simulink model "BPSK_Demod_OpenLoopClkRec_Prototype"  (R2013a)
settings: Solver=ode3  SolverMode=SingleTasking  StartTime=0.0  StopTime=10000/1200  FixedStep=1/480e3  RelTol=1e-3
undefined symbols (not defined in the file or in its folder): DiscIntNeverNeededParam
libraries: dsparch4 x9, simulink_extras x7, commsynccomp2 x6, dspsigops x6, simulink x5, commsink2 x2, commchan3 x1, commrflib2 x1, commrandsrc2 x1
settings Model: Creator=tibbs2010  LastModifiedBy=Cedric
settings DataIOCC: SignalLoggingSaveFormat=ModelDataLogs
settings DebuggingCC: MultiTaskDSMMsg=warning  MultiTaskCondExecSysMsg=none  StrictBusMsg=None
settings RTWCC: IncludeERTFirstTime=on

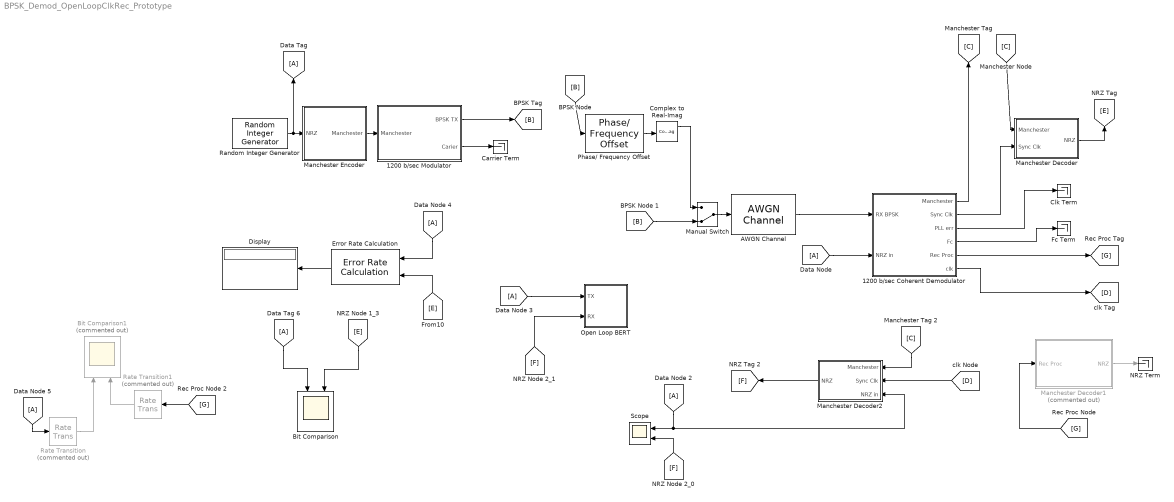
== system BPSK_Demod_OpenLoopClkRec_Prototype ==
  1200 b/sec Modulator : Subsystem
  1200 b/sec Coherent Demodulator : Subsystem
  AWGN Channel : commchan3/AWGN Channel  InputProcessing=Columns as channels (frame based)  seed=randseed  noiseMode="Signal to noise ratio  (Eb/No)"  EbNodB=0  EsNodB=10  SNRdB=10  bitsPerSym=1  Ps=12.5  Tsym=1/1200  variance=1
  Bit Comparison : Scope  NumInputPorts=2
      settings: YMin=-0.5~-0.5  YMax=1.5~1.5
  Bit Comparison1 : Scope  Commented=on  NumInputPorts=2
      settings: YMin=-0.5~-0.5  YMax=1.5~1.5  SaveName=ScopeData19
  Carrier Term : Terminator
  Clk Term : Terminator
  Complex to Real-Imag : ComplexToRealImag
  Display : Display
  Error Rate Calculation : commsink2/Error Rate Calculation  N=3  st_delay=0  cp_mode=Entire frame  subframe=[]  PMode=Port  WsName=ErrorVec  RsMode2=off  stop=off  numErr=100  maxBits=1e6
  Fc Term : Terminator
  Manchester Encoder : Subsystem
  Manchester Decoder : Subsystem
  Manchester Decoder1 : Subsystem  Commented=on
  Manchester Decoder2 : Subsystem
  Manual Switch : ManualSwitch  CurrentSetting=0
  NRZ Term : Terminator
  Open Loop BERT : Subsystem
  Phase/ Frequency Offset : commrflib2/Phase// Frequency Offset  phaseOffset=30  freqPort=off  freqOffset=0
  Random Integer Generator : commrandsrc2/Random Integer Generator  mul=2  seed=randseed  Ts=1/1200  frameBased=off  sampPerFrame=1  orient=off  outDataType=double
  Rate Transition : RateTransition  Commented=on  OutPortSampleTime=1/1200
  Rate Transition1 : RateTransition  Commented=on  OutPortSampleTime=1/1200
  Scope : Scope  NumInputPorts=2
      settings: YMin=-5~-5  YMax=5~5  SaveName=ScopeData26
  wires:
  Error Rate Calculation/1 -> Display/1
  1200 b/sec Coherent Demodulator/1(Manchester) -> [C]
  1200 b/sec Coherent Demodulator/2(Sync Clk) -> Manchester Decoder/2(Sync Clk)
  Phase/ Frequency Offset/1 -> Complex to Real-Imag/1
  Complex to Real-Imag/1 -> Manual Switch/1
  Manual Switch/1 -> AWGN Channel/1
  AWGN Channel/1 -> 1200 b/sec Coherent Demodulator/1(RX BPSK)
  1200 b/sec Coherent Demodulator/5(Rec Proc) -> [G]
  1200 b/sec Coherent Demodulator/3(PLL err) -> Clk Term/1
  1200 b/sec Coherent Demodulator/4(Fc) -> Fc Term/1
  Rate Transition/1 -> Bit Comparison1/1
  Rate Transition1/1 -> Bit Comparison1/2
  1200 b/sec Coherent Demodulator/6(clk) -> [D]
  [A] -> Open Loop BERT/1(TX)
  [B] -> Phase/ Frequency Offset/1
  [B] -> Manual Switch/2
  [A] -> 1200 b/sec Coherent Demodulator/2(NRZ in)
  [A] -> Rate Transition/1
  [A] -> Manchester Decoder2/3(NRZ in), Scope/1
  [A] -> Error Rate Calculation/1
  [A] -> Bit Comparison/1
  [C] -> Manchester Decoder/1(Manchester)
  [C] -> Manchester Decoder2/1(Manchester)
  [D] -> Manchester Decoder2/2(Sync Clk)
  Manchester Decoder/1(NRZ) -> [E]
  [E] -> Bit Comparison/2
  Manchester Decoder2/1(NRZ) -> [F]
  [G] -> Manchester Decoder1/1(Rec Proc)
  [G] -> Rate Transition1/1
  Manchester Decoder1/1(NRZ) -> NRZ Term/1
  [F] -> Open Loop BERT/2(RX)
  [F] -> Scope/2
  [E] -> Error Rate Calculation/2
  1200 b/sec Modulator/2(Carier) -> Carrier Term/1
  1200 b/sec Modulator/1(BPSK TX) -> [B]
  Random Integer Generator/1 -> Manchester Encoder/1(NRZ), [A]
  Manchester Encoder/1(Manchester) -> 1200 b/sec Modulator/1(Manchester)

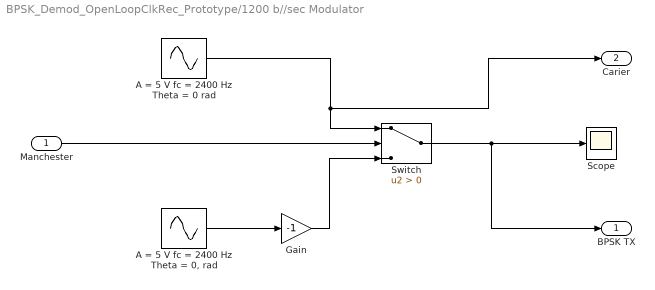
== system BPSK_Demod_OpenLoopClkRec_Prototype/1200 b//sec Modulator ==
  Manchester : Inport
  A = 5 V fc = 2400 Hz Theta = 0 rad : Sin  Amplitude=5  Frequency=2*pi*2400  Phase=pi/2  SampleTime=1/480e3
  "A = 5 V fc = 2400 Hz Theta = 0, rad" : Sin  Amplitude=5  Frequency=2*pi*2400  Phase=pi/2  SampleTime=1/480e3  Offset=pi
  Gain : Gain  Gain=-1
  Scope : Scope
      settings: SaveName=ScopeData22
  Switch : Switch  Criteria=u2 > Threshold
  BPSK TX : Outport
  Carier : Outport  Port=2
  wires:
  A = 5 V fc = 2400 Hz Theta = 0 rad/1 -> Switch/1, Carier/1
  "A = 5 V fc = 2400 Hz Theta = 0, rad"/1 -> Gain/1
  Gain/1 -> Switch/3
  Manchester/1 -> Switch/2
  Switch/1 -> Scope/1, BPSK TX/1

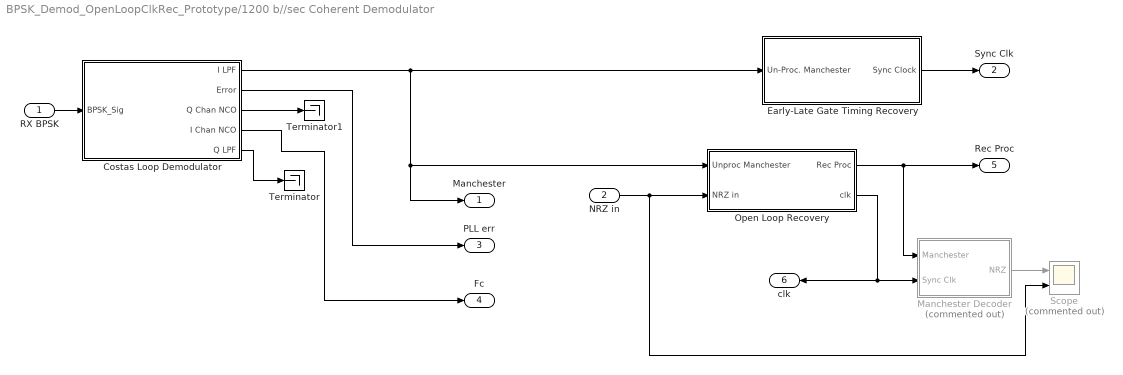
== system BPSK_Demod_OpenLoopClkRec_Prototype/1200 b//sec Coherent Demodulator ==
  RX BPSK : Inport
  NRZ in : Inport  Port=2
  Costas Loop Demodulator : Subsystem
  Early-Late Gate Timing Recovery : Subsystem
  Manchester Decoder : Subsystem  Commented=on
  Open Loop Recovery : Subsystem
  Scope : Scope  Commented=on  NumInputPorts=2
      settings: YMin=-5~-5  YMax=5~5  SaveName=ScopeData20
  Terminator : Terminator
  Terminator1 : Terminator
  Manchester : Outport
  Sync Clk : Outport  Port=2
  PLL err : Outport  Port=3
  Fc : Outport  Port=4
  Rec Proc : Outport  Port=5
  clk : Outport  Port=6
  wires:
  RX BPSK/1 -> Costas Loop Demodulator/1(BPSK_Sig)
  Early-Late Gate Timing Recovery/1(Sync Clock) -> Sync Clk/1
  Costas Loop Demodulator/2(Error) -> PLL err/1
  Costas Loop Demodulator/4(I Chan NCO) -> Fc/1
  Costas Loop Demodulator/1(I LPF) -> Manchester/1, Open Loop Recovery/1(Unproc Manchester), Early-Late Gate Timing Recovery/1(Un-Proc. Manchester)
  Open Loop Recovery/1(Rec Proc) -> Rec Proc/1, Manchester Decoder/1(Manchester)
  NRZ in/1 -> Scope/2, Open Loop Recovery/2(NRZ in)
  Open Loop Recovery/2(clk) -> Manchester Decoder/2(Sync Clk), clk/1
  Manchester Decoder/1(NRZ) -> Scope/1
  Costas Loop Demodulator/3(Q Chan NCO) -> Terminator1/1
  Costas Loop Demodulator/5(Q LPF) -> Terminator/1

== system BPSK_Demod_OpenLoopClkRec_Prototype/Manchester Encoder ==
  NRZ : Inport
  Logical Operator : Logic  Operator=XOR  IconShape=distinctive  AllPortsSameDT=off  OutDataTypeStr=boolean
  Rate Transition : RateTransition  OutPortSampleTime=1/480e3
  TX Clk : DiscretePulseGenerator  PulseType=Time based  Period=1/1200  PulseWidth=50
  Manchester : Outport
  wires:
  Rate Transition/1 -> Logical Operator/1
  Logical Operator/1 -> Manchester/1
  NRZ/1 -> Rate Transition/1
  TX Clk/1 -> Logical Operator/2

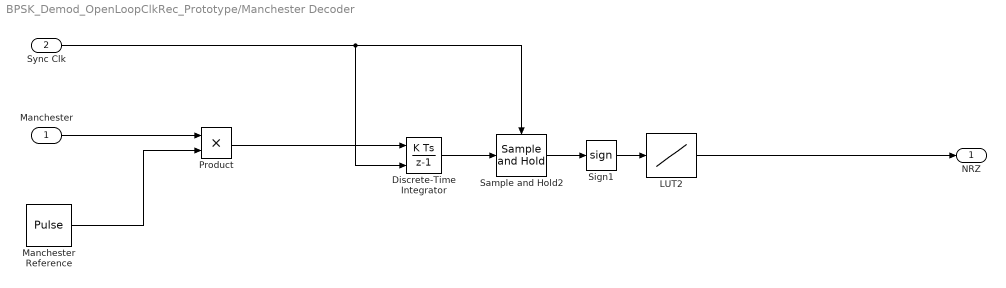
== system BPSK_Demod_OpenLoopClkRec_Prototype/Manchester Decoder ==
  Manchester : Inport
  Sync Clk : Inport  Port=2
  Discrete-Time Integrator : DiscreteIntegrator  ExternalReset=rising  SampleTime=1/480e3  ICPrevOutput=DiscIntNeverNeededParam  ICPrevScaledInput=DiscIntNeverNeededParam
  LUT2 : Lookup_n-D  NumberOfTableDimensions=1  BreakpointsForDimension1=[-1 0 1]  Table=[0 0 1]  RndMeth=Simplest  InputSameDT=on
  Manchester Reference : DiscretePulseGenerator  PulseType=Time based  Period=1/1200  PulseWidth=50  PhaseDelay=(1/1200)/2
  Product : Product
  Sample and Hold2 : dspsigops/Sample and Hold  trig=Falling edge  initCond=0  latchinput=off
  Sign1 : Signum
  NRZ : Outport
  wires:
  Discrete-Time Integrator/1 -> Sample and Hold2/1
  Sample and Hold2/1 -> Sign1/1
  Sign1/1 -> LUT2/1
  Manchester/1 -> Product/1
  Product/1 -> Discrete-Time Integrator/1
  LUT2/1 -> NRZ/1
  Sync Clk/1 -> Discrete-Time Integrator/2, Sample and Hold2/Trigger
  Manchester Reference/1 -> Product/2

== system BPSK_Demod_OpenLoopClkRec_Prototype/Manchester Decoder1 ==
  Rec Proc : Inport
  CDR : Subsystem
  ML decoder : Subsystem
  Scope : Scope  NumInputPorts=2
      settings: YMin=-0.5~-5  YMax=1.5~5  SaveName=ScopeData7
  Scope1 : Scope
      settings: YMin=-0.5  YMax=1.5  SaveName=ScopeData9
  NRZ : Outport
  wires:
  CDR/1(CLK) -> Scope/2, ML decoder/1(CLK)
  Rec Proc/1 -> ML decoder/2(Manchester), Scope/1, CDR/1(Edges)
  ML decoder/1(NRZ) -> NRZ/1, Scope1/1

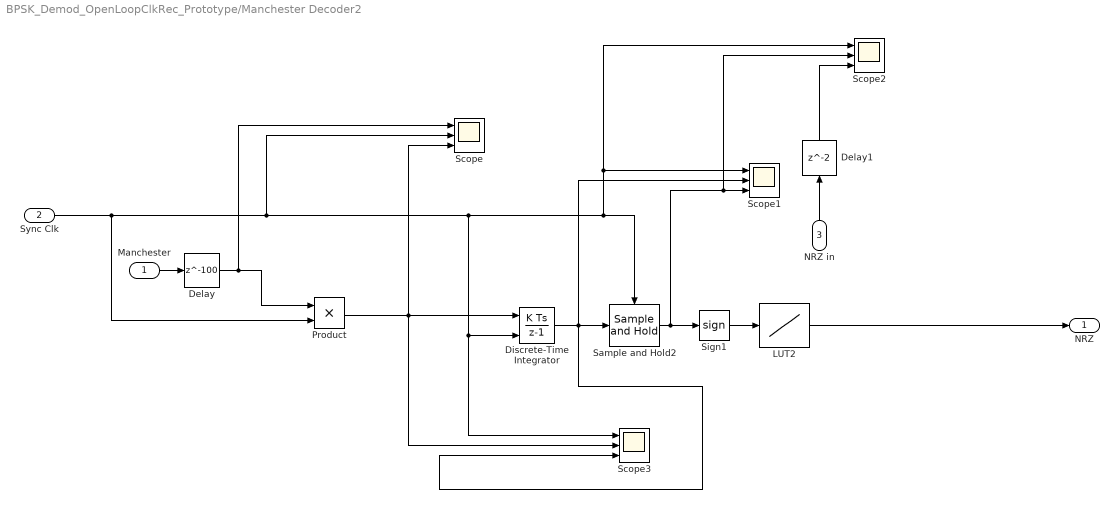
== system BPSK_Demod_OpenLoopClkRec_Prototype/Manchester Decoder2 ==
  Manchester : Inport
  Sync Clk : Inport  Port=2
  NRZ in : Inport  Port=3
  Delay : Delay  DelayLength=100  InitialCondition=0  SampleTime=1/480e3
  Delay1 : Delay  InitialCondition=0  SampleTime=1/1200
  Discrete-Time Integrator : DiscreteIntegrator  ExternalReset=rising  SampleTime=1/480e3  ICPrevOutput=DiscIntNeverNeededParam  ICPrevScaledInput=DiscIntNeverNeededParam
  LUT2 : Lookup_n-D  NumberOfTableDimensions=1  BreakpointsForDimension1=[-1 0 1]  Table=[1 1 0]  RndMeth=Simplest  InputSameDT=on
  Product : Product
  Sample and Hold2 : dspsigops/Sample and Hold  trig=Falling edge  initCond=0  latchinput=off
  Scope{,1..3} (4 alike) : Scope  NumInputPorts=3
      Scope settings: YMin=-4.5~0~-4.5  YMax=3.5~1~3.5  SaveName=ScopeData21
      Scope1 settings: YMin=-5~-5~-5  YMax=5~5~5  SaveName=ScopeData25
      Scope2 settings: YMin=-5~-5~-5  YMax=5~5~5  SaveName=ScopeData27
      Scope3 settings: YMin=-5~-5~-5  YMax=5~5~5  SaveName=ScopeData28
  Sign1 : Signum
  NRZ : Outport
  wires:
  Discrete-Time Integrator/1 -> Scope3/3, Scope1/2, Sample and Hold2/1
  Sample and Hold2/1 -> Scope2/2, Scope1/3, Sign1/1
  Sign1/1 -> LUT2/1
  Manchester/1 -> Delay/1
  Product/1 -> Scope3/2, Scope/3, Discrete-Time Integrator/1
  LUT2/1 -> NRZ/1
  Sync Clk/1 -> Scope3/1, Discrete-Time Integrator/2, Scope1/1, Scope2/1, Sample and Hold2/Trigger, Scope/2, Product/2
  Delay/1 -> Scope/1, Product/1
  NRZ in/1 -> Delay1/1
  Delay1/1 -> Scope2/3

== system BPSK_Demod_OpenLoopClkRec_Prototype/Open Loop BERT ==
  note: SNR - BER
      | 15 - 0
      | 10 - 0.0040004
      | 8 - 0.0153
      | 6 - 0.04847
      | 4 - 0.1517
      | 2 - 0.2188
      | 0 - 0.3488
  TX : Inport
  RX : Inport  Port=2
  Bit Comparison : Scope  NumInputPorts=2
      settings: YMin=-0.5~-0.5  YMax=1.5~1.5  SaveName=ScopeData2
  Delay : Delay  InitialCondition=0  SampleTime=1/1200
  Display : Display
  Error Rate Calculation : commsink2/Error Rate Calculation  N=2  st_delay=0  cp_mode=Entire frame  subframe=[]  PMode=Port  WsName=ErrorVec  RsMode2=off  stop=off  numErr=100  maxBits=1e6
  Rate Transition1 : RateTransition  OutPortSampleTime=1/1200
  wires:
  RX/1 -> Rate Transition1/1
  TX/1 -> Error Rate Calculation/1, Delay/1
  Error Rate Calculation/1 -> Display/1
  Rate Transition1/1 -> Bit Comparison/2, Error Rate Calculation/2
  Delay/1 -> Bit Comparison/1

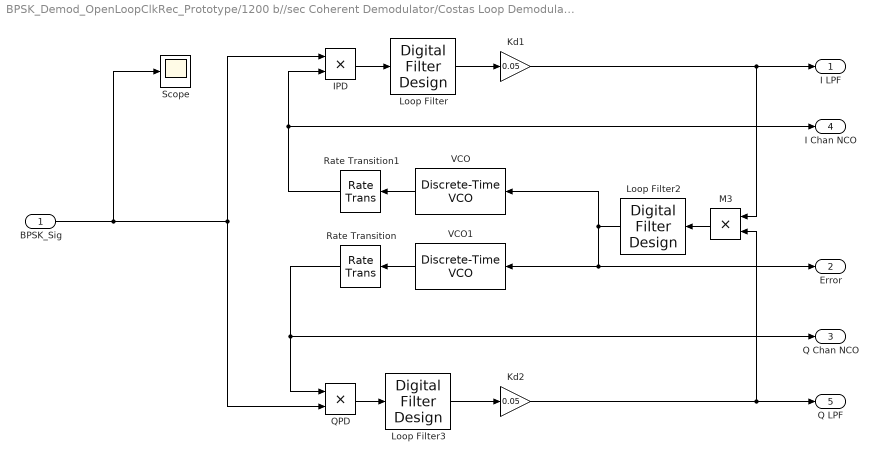
== system BPSK_Demod_OpenLoopClkRec_Prototype/1200 b//sec Coherent Demodulator/Costas Loop Demodulator ==
  BPSK_Sig : Inport
  IPD : Product
  Kd1 : Gain  Gain=0.05
  Kd2 : Gain  Gain=0.05
  Loop Filter : dsparch4/Digital Filter Design  mwdsp_browser_bugfix_var=off
  Loop Filter2 : dsparch4/Digital Filter Design  mwdsp_browser_bugfix_var=off
  Loop Filter3 : dsparch4/Digital Filter Design  mwdsp_browser_bugfix_var=off
  M3 : Product
  QPD : Product
  Rate Transition : RateTransition  OutPortSampleTime=1/480e3
  Rate Transition1 : RateTransition  OutPortSampleTime=1/480e3
  Scope : Scope
      settings: SaveName=ScopeData23
  VCO : commsynccomp2/Discrete-Time VCO  Ac=5  Fc=2400  Kc=.5  Ph=0  ts=1/480e3
  VCO1 : commsynccomp2/Discrete-Time VCO  Ac=5  Fc=2400  Kc=.5  Ph=pi/2  ts=1/480e3
  I LPF : Outport
  Error : Outport  Port=2
  Q Chan NCO : Outport  Port=3
  I Chan NCO : Outport  Port=4
  Q LPF : Outport  Port=5
  wires:
  VCO/1 -> Rate Transition1/1
  VCO1/1 -> Rate Transition/1
  Loop Filter3/1 -> Kd2/1
  QPD/1 -> Loop Filter3/1
  Rate Transition/1 -> QPD/1, Q Chan NCO/1
  Rate Transition1/1 -> IPD/2, I Chan NCO/1
  IPD/1 -> Loop Filter/1
  Loop Filter/1 -> Kd1/1
  M3/1 -> Loop Filter2/1
  Loop Filter2/1 -> VCO/1, Error/1, VCO1/1
  Kd2/1 -> Q LPF/1, M3/2
  Kd1/1 -> I LPF/1, M3/1
  BPSK_Sig/1 -> Scope/1, IPD/1, QPD/2

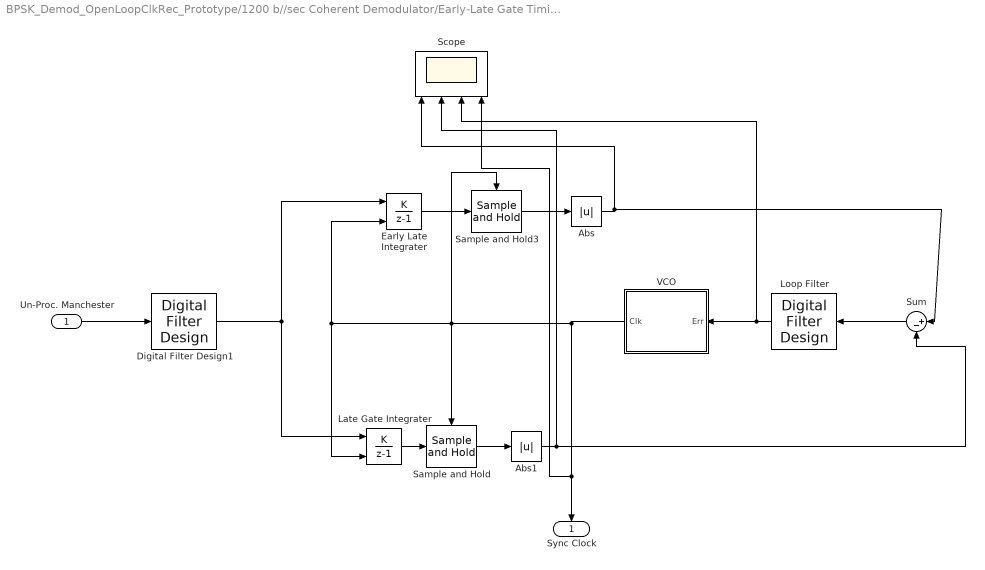
== system BPSK_Demod_OpenLoopClkRec_Prototype/1200 b//sec Coherent Demodulator/Early-Late Gate Timing Recovery ==
  Un-Proc. Manchester : Inport
  Abs : Abs
  Abs1 : Abs
  Digital Filter Design1 : dsparch4/Digital Filter Design  mwdsp_browser_bugfix_var=off
  Early Late Integrater : DiscreteIntegrator  IntegratorMethod=Accumulation: Forward Euler  ExternalReset=rising  SampleTime=1/480e3  ICPrevOutput=DiscIntNeverNeededParam  ICPrevScaledInput=DiscIntNeverNeededParam
  Late Gate Integrater : DiscreteIntegrator  IntegratorMethod=Accumulation: Forward Euler  ExternalReset=falling  SampleTime=1/480e3  ICPrevOutput=DiscIntNeverNeededParam  ICPrevScaledInput=DiscIntNeverNeededParam
  Loop Filter : dsparch4/Digital Filter Design  mwdsp_browser_bugfix_var=off
  Sample and Hold : dspsigops/Sample and Hold  trig=Rising edge  initCond=0  latchinput=off
  Sample and Hold3 : dspsigops/Sample and Hold  trig=Falling edge  initCond=0  latchinput=off
  Scope : Scope  NumInputPorts=4
      settings: YMin=0~0~-3000~-5  YMax=3500~3250~3000~5  SaveName=ScopeData4
  Sum : Sum  Inputs=|+-
  VCO : Subsystem
  Sync Clock : Outport
  wires:
  Abs/1 -> Sum/1, Scope/1
  Abs1/1 -> Sum/2, Scope/2
  Un-Proc. Manchester/1 -> Digital Filter Design1/1
  VCO/1(Clk) -> Scope/4, Sync Clock/1, Sample and Hold3/Trigger, Sample and Hold/Trigger, Late Gate Integrater/2, Early Late Integrater/2
  Sample and Hold/1 -> Abs1/1
  Late Gate Integrater/1 -> Sample and Hold/1
  Early Late Integrater/1 -> Sample and Hold3/1
  Sample and Hold3/1 -> Abs/1
  Loop Filter/1 -> Scope/3, VCO/1(Err)
  Sum/1 -> Loop Filter/1
  Digital Filter Design1/1 -> Late Gate Integrater/1, Early Late Integrater/1

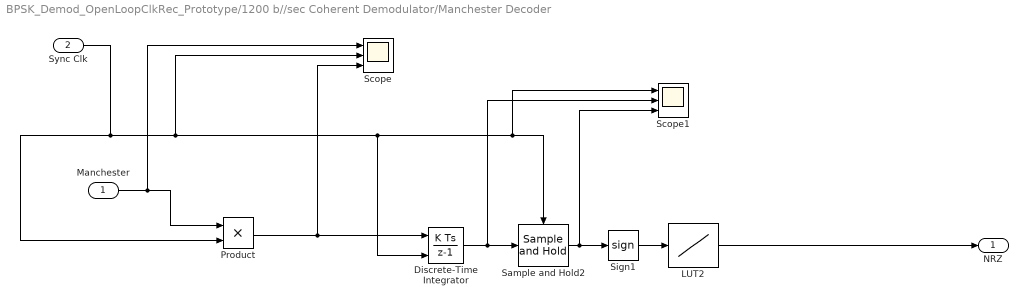
== system BPSK_Demod_OpenLoopClkRec_Prototype/1200 b//sec Coherent Demodulator/Manchester Decoder ==
  Manchester : Inport
  Sync Clk : Inport  Port=2
  Discrete-Time Integrator : DiscreteIntegrator  ExternalReset=rising  SampleTime=1/480e3  ICPrevOutput=DiscIntNeverNeededParam  ICPrevScaledInput=DiscIntNeverNeededParam
  LUT2 : Lookup_n-D  NumberOfTableDimensions=1  BreakpointsForDimension1=[-1 0 1]  Table=[1 1 0]  RndMeth=Simplest  InputSameDT=on
  Product : Product
  Sample and Hold2 : dspsigops/Sample and Hold  trig=Falling edge  initCond=0  latchinput=off
  Scope : Scope  NumInputPorts=3
      settings: YMin=-5~-5~-5  YMax=5~5~5  SaveName=ScopeData21
  Scope1 : Scope  NumInputPorts=3
      settings: YMin=-5~-5~-5  YMax=5~5~5  SaveName=ScopeData25
  Sign1 : Signum
  NRZ : Outport
  wires:
  Discrete-Time Integrator/1 -> Scope1/2, Sample and Hold2/1
  Sample and Hold2/1 -> Scope1/3, Sign1/1
  Sign1/1 -> LUT2/1
  Manchester/1 -> Scope/1, Product/1
  Product/1 -> Scope/3, Discrete-Time Integrator/1
  LUT2/1 -> NRZ/1
  Sync Clk/1 -> Discrete-Time Integrator/2, Scope1/1, Sample and Hold2/Trigger, Scope/2, Product/2

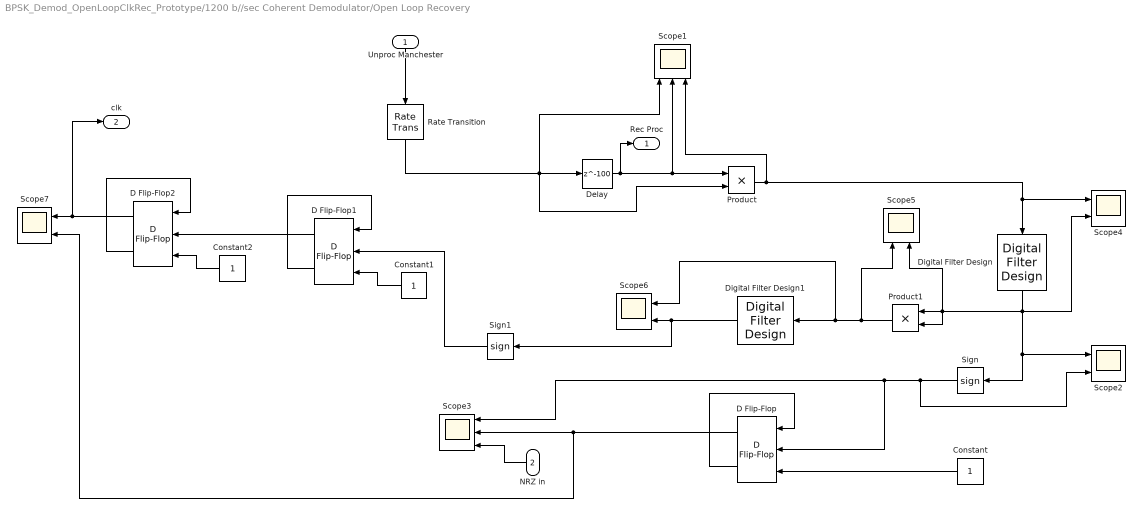
== system BPSK_Demod_OpenLoopClkRec_Prototype/1200 b//sec Coherent Demodulator/Open Loop Recovery ==
  Unproc Manchester : Inport
  NRZ in : Inport  Port=2
  Constant : Constant
  Constant1 : Constant
  Constant2 : Constant
  D Flip-Flop : simulink_extras/Flip Flops/D Flip-Flop
  D Flip-Flop1 : simulink_extras/Flip Flops/D Flip-Flop
  D Flip-Flop2 : simulink_extras/Flip Flops/D Flip-Flop
  Delay : Delay  DelayLength=100  InitialCondition=0  SampleTime=1/480e3
  Digital Filter Design : dsparch4/Digital Filter Design  mwdsp_browser_bugfix_var=off
  Digital Filter Design1 : dsparch4/Digital Filter Design  mwdsp_browser_bugfix_var=off
  Product : Product  SampleTime=1/480e3
  Product1 : Product  SampleTime=1/480e3
  Rate Transition : RateTransition  OutPortSampleTime=1/480e3
  Scope1 : Scope  NumInputPorts=3
      settings: YMin=-5~-5~-5  YMax=5~5~5  SaveName=ScopeData5
  Scope{2,4..7} (5 alike) : Scope  NumInputPorts=2
      Scope2 settings: YMin=-5~-5  YMax=5~5  SaveName=ScopeData6
      Scope4 settings: YMin=-5~-5  YMax=5~5  SaveName=ScopeData14
      Scope5 settings: YMin=-5~-5  YMax=5~5  SaveName=ScopeData29
      Scope6 settings: YMin=-5~-5  YMax=5~5  SaveName=ScopeData30
      Scope7 settings: YMin=-5~-5  YMax=5~5  SaveName=ScopeData31
  Scope3 : Scope  NumInputPorts=3
      settings: TimeRange=0.09  YMin=-1~0~-1  YMax=1~1~1  SaveName=ScopeData3
  Sign : Signum
  Sign1 : Signum
  Rec Proc : Outport
  clk : Outport  Port=2
  wires:
  Digital Filter Design/1 -> Scope4/2, Product1/1, Scope5/2, Product1/2, Scope2/1, Sign/1
  Delay/1 -> Rec Proc/1, Product/1, Scope1/2
  Constant/1 -> D Flip-Flop/3
  Sign/1 -> Scope2/2, D Flip-Flop/2, Scope3/1
  D Flip-Flop/2 -> D Flip-Flop/1
  Unproc Manchester/1 -> Rate Transition/1
  Rate Transition/1 -> Scope1/1, Product/2, Delay/1
  Product/1 -> Scope4/1, Digital Filter Design/1, Scope1/3
  D Flip-Flop/1 -> Scope7/2, Scope3/2
  NRZ in/1 -> Scope3/3
  Product1/1 -> Scope6/1, Digital Filter Design1/1, Scope5/1
  Digital Filter Design1/1 -> Sign1/1, Scope6/2
  Constant1/1 -> D Flip-Flop1/3
  Sign1/1 -> D Flip-Flop1/2
  D Flip-Flop1/2 -> D Flip-Flop1/1
  Constant2/1 -> D Flip-Flop2/3
  D Flip-Flop1/1 -> D Flip-Flop2/2
  D Flip-Flop2/2 -> D Flip-Flop2/1
  D Flip-Flop2/1 -> clk/1, Scope7/1

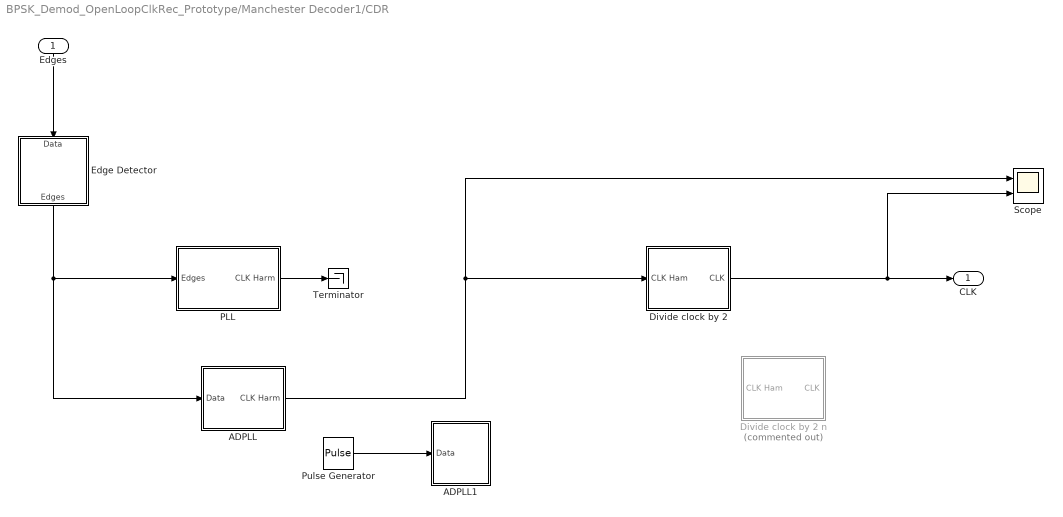
== system BPSK_Demod_OpenLoopClkRec_Prototype/Manchester Decoder1/CDR ==
  Edges : Inport
  ADPLL : Subsystem
  ADPLL1 : Subsystem
  Divide clock by 2 : Subsystem
  Divide clock by 2 n : Subsystem  Commented=on
  Edge Detector : Subsystem
  PLL : Subsystem
  Pulse Generator : DiscretePulseGenerator  Amplitude=-1  Period=2200  PulseWidth=600  SampleTime=1/480e3
  Scope : Scope  NumInputPorts=2
      settings: YMin=-0.5~-5  YMax=1.5~5  SaveName=ScopeData8
  Terminator : Terminator
  CLK : Outport
  wires:
  Edge Detector/1(Edges) -> ADPLL/1(Data), PLL/1(Edges)
  Edges/1 -> Edge Detector/1(Data)
  Divide clock by 2/1(CLK) -> Scope/2, CLK/1
  Pulse Generator/1 -> ADPLL1/1(Data)
  ADPLL/1(CLK Harm) -> Scope/1, Divide clock by 2/1(CLK Ham)
  PLL/1(CLK Harm) -> Terminator/1

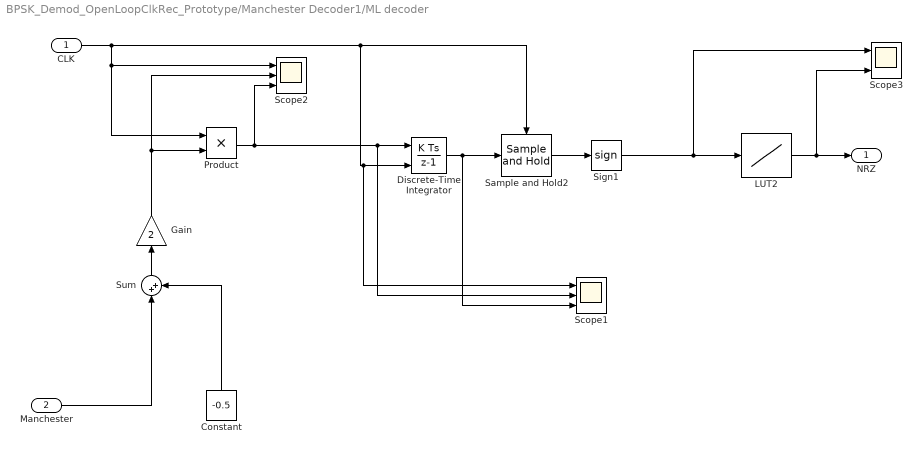
== system BPSK_Demod_OpenLoopClkRec_Prototype/Manchester Decoder1/ML decoder ==
  CLK : Inport
  Manchester : Inport  Port=2
  Constant : Constant  Value=-0.5
  Discrete-Time Integrator : DiscreteIntegrator  ExternalReset=rising  SampleTime=1/480e3  ICPrevOutput=DiscIntNeverNeededParam  ICPrevScaledInput=DiscIntNeverNeededParam
  Gain : Gain  Gain=2
  LUT2 : Lookup_n-D  NumberOfTableDimensions=1  BreakpointsForDimension1=[-1 0 1]  Table=[1 1 0]  RndMeth=Simplest  InputSameDT=on
  Product : Product
  Sample and Hold2 : dspsigops/Sample and Hold  trig=Falling edge  initCond=0  latchinput=off
  Scope1 : Scope  NumInputPorts=3
      settings: YMin=-0.5~-5~-5  YMax=1.5~5~5  SaveName=ScopeData10
  Scope2 : Scope  NumInputPorts=3
      settings: YMin=-0.5~-5~-5  YMax=1.5~5~5  SaveName=ScopeData11
  Scope3 : Scope  NumInputPorts=2
      settings: YMin=-1.5~-0.5  YMax=1.5~1.5  SaveName=ScopeData12
  Sign1 : Signum
  Sum : Sum  Inputs=|++
  NRZ : Outport
  wires:
  Product/1 -> Scope2/3, Scope1/2, Discrete-Time Integrator/1
  CLK/1 -> Product/1, Scope2/1, Scope1/1, Discrete-Time Integrator/2, Sample and Hold2/Trigger
  Sample and Hold2/1 -> Sign1/1
  Discrete-Time Integrator/1 -> Scope1/3, Sample and Hold2/1
  Sign1/1 -> Scope3/1, LUT2/1
  Manchester/1 -> Sum/1
  Sum/1 -> Gain/1
  Gain/1 -> Scope2/2, Product/2
  Constant/1 -> Sum/2
  LUT2/1 -> Scope3/2, NRZ/1

== system BPSK_Demod_OpenLoopClkRec_Prototype/1200 b//sec Coherent Demodulator/Early-Late Gate Timing Recovery/VCO ==
  Err : Inport
  Discrete-Time VCO : commsynccomp2/Discrete-Time VCO  Ac=1  Fc=1200  Kc=0.15  Ph=pi/2  ts=1/480e3
  LUT1 : Lookup_n-D  NumberOfTableDimensions=1  BreakpointsForDimension1=[-1 0 1]  Table=[0 0 1]  RndMeth=Simplest  InputSameDT=on
  Rate Transition2 : RateTransition  OutPortSampleTime=1/480e3
  Sign : Signum
  Clk : Outport
  wires:
  Discrete-Time VCO/1 -> Sign/1
  Err/1 -> Discrete-Time VCO/1
  LUT1/1 -> Rate Transition2/1
  Rate Transition2/1 -> Clk/1
  Sign/1 -> LUT1/1

== system BPSK_Demod_OpenLoopClkRec_Prototype/Manchester Decoder1/CDR/ADPLL ==
  Data : Inport
  Hogge : Subsystem
  Loop Filter : dsparch4/Digital Filter Design  mwdsp_browser_bugfix_var=off
  NCO : Subsystem
  Rate Transition : RateTransition  OutPortSampleTime=1/480e3
  Scope : Scope  NumInputPorts=2
      settings: YMin=-1~-0.475  YMax=0~-0.225  SaveName=ScopeData5
  CLK Harm : Outport
  wires:
  Data/1 -> Hogge/1(Data)
  Loop Filter/1 -> Scope/2, NCO/1(error)
  Hogge/1(Edges) -> Rate Transition/1, Scope/1
  Rate Transition/1 -> Loop Filter/1
  NCO/1(Pulses) -> Hogge/2(CLK VCO), CLK Harm/1

== system BPSK_Demod_OpenLoopClkRec_Prototype/Manchester Decoder1/CDR/ADPLL1 ==
  Data : Inport
  NCO : Subsystem
  wires:
  Data/1 -> NCO/1(error)

== system BPSK_Demod_OpenLoopClkRec_Prototype/Manchester Decoder1/CDR/Divide clock by 2 ==
  CLK Ham : Inport
  Constant : Constant
  D Flip-Flop : simulink_extras/Flip Flops/D Flip-Flop
  CLK : Outport
  wires:
  Constant/1 -> D Flip-Flop/3
  D Flip-Flop/2 -> D Flip-Flop/1
  CLK Ham/1 -> D Flip-Flop/2
  D Flip-Flop/1 -> CLK/1

== system BPSK_Demod_OpenLoopClkRec_Prototype/Manchester Decoder1/CDR/Divide clock by 2 n ==
  CLK Ham : Inport
  Constant : Constant
  D Flip-Flop : simulink_extras/Flip Flops/D Flip-Flop
  CLK : Outport
  wires:
  Constant/1 -> D Flip-Flop/3
  D Flip-Flop/2 -> D Flip-Flop/1
  CLK Ham/1 -> D Flip-Flop/2
  D Flip-Flop/1 -> CLK/1

== system BPSK_Demod_OpenLoopClkRec_Prototype/Manchester Decoder1/CDR/Edge Detector ==
  Data : Inport
  Data Type Conversion1 : DataTypeConversion
  Delay : Delay  DelayLength=100  InitialCondition=0
  Scope : Scope  NumInputPorts=3
      settings: YMin=-5~-5~-5  YMax=5~5~5
  XOR1 : Logic  Operator=XOR  IconShape=distinctive  AllPortsSameDT=off  OutDataTypeStr=boolean
  Edges : Outport
  wires:
  Delay/1 -> XOR1/2, Scope/2
  XOR1/1 -> Scope/3, Data Type Conversion1/1
  Data/1 -> XOR1/1, Delay/1, Scope/1
  Data Type Conversion1/1 -> Edges/1

== system BPSK_Demod_OpenLoopClkRec_Prototype/Manchester Decoder1/CDR/PLL ==
  Edges : Inport
  Compare : simulink/Logic and Bit Operations/Compare To Constant  relop=>  const=0  OutDataTypeStr=boolean
  Scope1 : Scope  NumInputPorts=4
      settings: YMin=0~0~0~0  YMax=1~1~1~650
  Scope2 : Scope
      settings: YMin=-0.5  YMax=1.5  SaveName=ScopeData13
  VCO : Subsystem
  XOR : Logic  Operator=XOR  IconShape=distinctive  AllPortsSameDT=off  OutDataTypeStr=boolean
  CLK Harm : Outport
  wires:
  XOR/1 -> VCO/1(Edges), Scope1/3
  VCO/1(Error) -> Scope1/4
  VCO/2(Output VCO) -> Compare/1, Scope2/1
  Edges/1 -> XOR/2, Scope1/1
  Compare/1 -> CLK Harm/1, XOR/1, Scope1/2

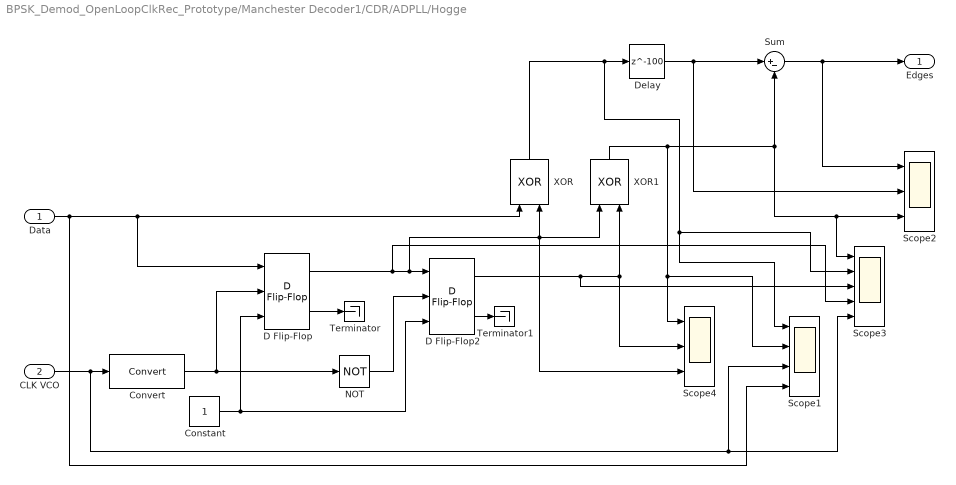
== system BPSK_Demod_OpenLoopClkRec_Prototype/Manchester Decoder1/CDR/ADPLL/Hogge ==
  Data : Inport
  CLK VCO : Inport  Port=2
  Constant : Constant  OutDataTypeStr=boolean  SampleTime=1/(19200)
  Convert : DataTypeConversion
  D Flip-Flop : simulink_extras/Flip Flops/D Flip-Flop
  D Flip-Flop2 : simulink_extras/Flip Flops/D Flip-Flop
  Delay : Delay  DelayLength=100  InitialCondition=0  SampleTime=1/480e3
  NOT : Logic  Operator=NOT  IconShape=distinctive  AllPortsSameDT=off  OutDataTypeStr=boolean
  Scope1 : Scope  NumInputPorts=4
      settings: YMin=-5~-5~-5~-5  YMax=5~5~5~5  SaveName=ScopeData16
  Scope2 : Scope  NumInputPorts=3
      settings: YMin=-5~-5~-5  YMax=5~5~5  SaveName=ScopeData2
  Scope3 : Scope  NumInputPorts=5
      settings: YMin=-5~-5~-5~-5~-5  YMax=5~5~5~5~5  SaveName=ScopeData17
  Scope4 : Scope  NumInputPorts=3
      settings: YMin=-5~-5~-5  YMax=5~5~5  SaveName=ScopeData18
  Sum : Sum  Inputs=|+-  OutDataTypeStr=double  SampleTime=1/4800
  Terminator : Terminator
  Terminator1 : Terminator
  XOR : Logic  Operator=XOR  IconShape=distinctive  AllPortsSameDT=off  OutDataTypeStr=boolean
  XOR1 : Logic  Operator=XOR  IconShape=distinctive  AllPortsSameDT=off  OutDataTypeStr=boolean
  Edges : Outport
  wires:
  NOT/1 -> D Flip-Flop2/2
  Constant/1 -> D Flip-Flop2/3, D Flip-Flop/3
  Convert/1 -> NOT/1, D Flip-Flop/2
  D Flip-Flop2/1 -> Scope3/3, Scope4/2, XOR1/2
  D Flip-Flop/1 -> Scope3/4, XOR/2, XOR1/1, Scope4/3, D Flip-Flop2/1
  D Flip-Flop/2 -> Terminator/1
  D Flip-Flop2/2 -> Terminator1/1
  Sum/1 -> Edges/1, Scope2/1
  XOR1/1 -> Scope4/1, Scope1/2, Scope3/1, Scope2/3, Sum/2
  CLK VCO/1 -> Scope3/5, Scope1/3, Convert/1
  Delay/1 -> Scope2/2, Sum/1
  Data/1 -> Scope1/4, XOR/1, D Flip-Flop/1
  XOR/1 -> Scope3/2, Scope1/1, Delay/1

== system BPSK_Demod_OpenLoopClkRec_Prototype/Manchester Decoder1/CDR/ADPLL/NCO ==
  error : Inport
  Continuous-Time VCO : commsynccomp2/Continuous-Time VCO  Ac=1  Fc=4800  Kc=1  Ph=0
  Gain : Gain  Gain=5e3
  Greater : simulink/Logic and Bit Operations/Compare To Zero  relop=>  OutDataTypeStr=boolean
  PID Controller : simulink/Continuous/PID Controller  Controller=PI  TimeDomain=Continuous-time  SampleTime=1  IntegratorMethod=Forward Euler  FilterMethod=Forward Euler  Form=Parallel  P=0.5  I=0  D=200  N=2  InitialConditionSource=internal  InitialConditionForIntegrator=0  InitialConditionForFilter=0  ExternalReset=none  LimitOutput=on  UpperSaturationLimit=4800  LowerSaturationLimit=-4800  LinearizeAsGain=on  AntiWindupMode=none  Kb=1  TrackingMode=off  Kt=1  PParamMin=[]  PParamMax=[]  IParamMin=[]  IParamMax=[]  DParamMin=[]  DParamMax=[]  NParamMin=[]  NParamMax=[]  KbParamMin=[]  KbParamMax=[]  KtParamMin=[]  KtParamMax=[]  POutMin=[]  POutMax=[]  IOutMin=[]  IOutMax=[]  DOutMin=[]  DOutMax=[]  NOutMin=[]  NOutMax=[]  KbOutMin=[]  KbOutMax=[]  KtOutMin=[]  KtOutMax=[]  IntegratorOutMin=[]  IntegratorOutMax=[]  FilterOutMin=[]  FilterOutMax=[]  SumOutMin=[]  SumOutMax=[]  SumI1OutMin=[]  SumI1OutMax=[]  SumI2OutMin=[]  SumI2OutMax=[]  SumI3OutMin=[]  SumI3OutMax=[]  SumDOutMin=[]  SumDOutMax=[]  SaturationOutMin=[]  SaturationOutMax=[]  IntegratorContinuousStateAttributes=''  IntegratorStateMustResolveToSignalObject=off  IntegratorRTWStateStorageClass=Auto  FilterContinuousStateAttributes=''  FilterStateMustResolveToSignalObject=off  FilterRTWStateStorageClass=Auto
  Scope : Scope  NumInputPorts=3
      settings: YMin=-1250~-1~0  YMax=1000~1~1  SaveName=ScopeData4
  Scope1 : Scope  NumInputPorts=2
      settings: YMin=-1500~-3000  YMax=1500~2750  SaveName=ScopeData24
  Pulses : Outport
  wires:
  Greater/1 -> Scope/3, Pulses/1
  Continuous-Time VCO/1 -> Scope/2, Greater/1
  error/1 -> Gain/1
  Gain/1 -> Scope1/2, PID Controller/1
  PID Controller/1 -> Scope1/1, Continuous-Time VCO/1, Scope/1

== system BPSK_Demod_OpenLoopClkRec_Prototype/Manchester Decoder1/CDR/ADPLL1/NCO ==
  error : Inport
  Greater : simulink/Logic and Bit Operations/Compare To Zero  relop=<  OutDataTypeStr=boolean
  Rate Transition : RateTransition  OutPortSampleTime=1/480e3
  Scope : Scope  NumInputPorts=3
      settings: YMin=-1~-1~-5  YMax=0~1~5  SaveName=ScopeData4
  VCO : commsynccomp2/Discrete-Time VCO  Ac=1  Fc=1200  Kc=1000  Ph=0  ts=1/480e3
  wires:
  Greater/1 -> Scope/3
  VCO/1 -> Scope/2, Greater/1
  error/1 -> Rate Transition/1
  Rate Transition/1 -> Scope/1, VCO/1

== system BPSK_Demod_OpenLoopClkRec_Prototype/Manchester Decoder1/CDR/PLL/VCO ==
  Edges : Inport
  Convert : DataTypeConversion
  Discrete PID Controller : simulink/Continuous/PID Controller  Controller=PI  TimeDomain=Discrete-time  SampleTime=1/480e3  IntegratorMethod=Forward Euler  FilterMethod=Forward Euler  Form=Parallel  P=1200  I=0.5  D=0  N=2  InitialConditionSource=internal  InitialConditionForIntegrator=0  InitialConditionForFilter=0  ExternalReset=none  LimitOutput=off  UpperSaturationLimit=inf  LowerSaturationLimit=-inf  LinearizeAsGain=off  AntiWindupMode=none  Kb=1  TrackingMode=off  Kt=1  PParamMin=[]  PParamMax=[]  IParamMin=[]  IParamMax=[]  DParamMin=[]  DParamMax=[]  NParamMin=[]  NParamMax=[]  KbParamMin=[]  KbParamMax=[]  KtParamMin=[]  KtParamMax=[]  POutMin=[]  POutMax=[]  IOutMin=[]  IOutMax=[]  DOutMin=[]  DOutMax=[]  NOutMin=[]  NOutMax=[]  KbOutMin=[]  KbOutMax=[]  KtOutMin=[]  KtOutMax=[]  IntegratorOutMin=[]  IntegratorOutMax=[]  FilterOutMin=[]  FilterOutMax=[]  SumOutMin=[]  SumOutMax=[]  SumI1OutMin=[]  SumI1OutMax=[]  SumI2OutMin=[]  SumI2OutMax=[]  SumI3OutMin=[]  SumI3OutMax=[]  SumDOutMin=[]  SumDOutMax=[]  SaturationOutMin=[]  SaturationOutMax=[]  IntegratorContinuousStateAttributes=''  IntegratorStateMustResolveToSignalObject=off  IntegratorRTWStateStorageClass=Auto  FilterContinuousStateAttributes=''  FilterStateMustResolveToSignalObject=off  FilterRTWStateStorageClass=Auto
  Low- Pass : dsparch4/Digital Filter Design  Commented=on  mwdsp_browser_bugfix_var=off
  Scope : Scope
      settings: SaveName=ScopeData15
  VCO : commsynccomp2/Discrete-Time VCO  Ac=1  Fc=2400  Kc=4800  Ph=pi/2  ts=1/480e3
  Error : Outport
  Output VCO : Outport  Port=2
  wires:
  VCO/1 -> Output VCO/1
  Edges/1 -> Convert/1
  Discrete PID Controller/1 -> Scope/1, Error/1, VCO/1
  Convert/1 -> Discrete PID Controller/1
